simulink model "Position"  (R2020b)
settings: Solver=VariableStepAuto  StartTime=0.0  StopTime=10.0  RelTol=1e-3
values from neighbouring files (symbols this model uses):
  b = 3.5077E-6    [data.sldd]
  J = 3.228E-6    [data.sldd]
  L = 2.75E-6    [data.sldd]
  R = 4.0    [data.sldd]
undefined symbols (not defined in the file or in its folder): K
settings Model: Creator=smart  LastModifiedBy=smart

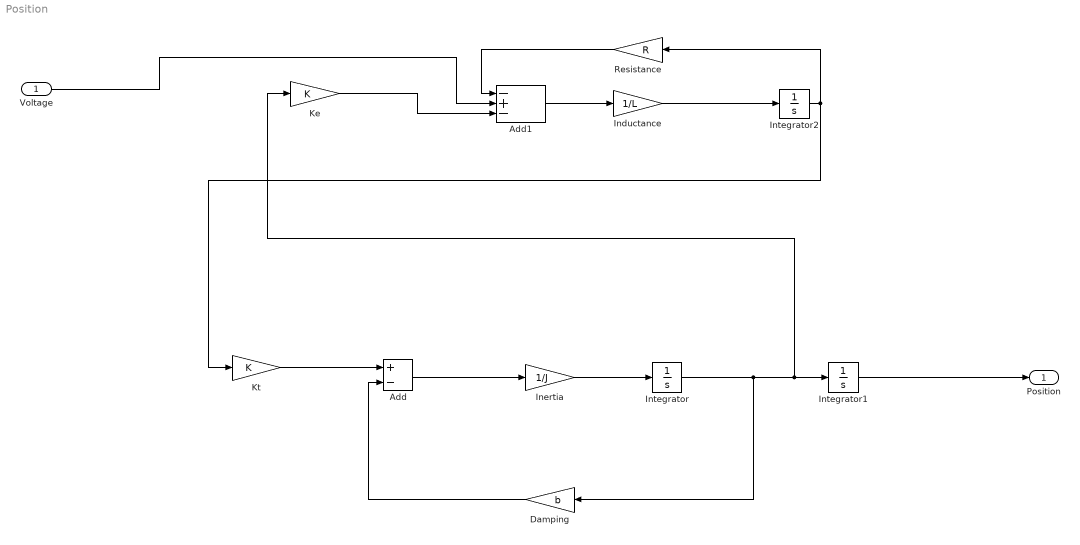
== system Position ==
  Voltage : Inport
  Add : Sum  Inputs=+-
  Add1 : Sum  Inputs=-+-
  Damping : Gain  Gain=b
  Inductance : Gain  Gain=1/L
  Inertia : Gain  Gain=1/J
  Integrator : Integrator
  Integrator1 : Integrator
  Integrator2 : Integrator
  Ke : Gain  Gain=K
  Kt : Gain  Gain=K
  Resistance : Gain  Gain=R
  Position : Outport
  wires:
  Kt/1 -> Add/1
  Add/1 -> Inertia/1
  Inertia/1 -> Integrator/1
  Integrator/1 -> Damping/1, Ke/1, Integrator1/1
  Integrator1/1 -> Position/1
  Damping/1 -> Add/2
  Ke/1 -> Add1/3
  Voltage/1 -> Add1/2
  Resistance/1 -> Add1/1
  Integrator2/1 -> Kt/1, Resistance/1
  Add1/1 -> Inductance/1
  Inductance/1 -> Integrator2/1
